simulink model "Hardware_With_Lead_Compensator"  (R2024b)
settings: Solver=FixedStepDiscrete  StartTime=0.0  StopTime=60  FixedStep=0.01  RelTol=1e-3  EnableMultiTasking=on
model workspace (MAT data in the model file):
  Kd = 0
  Ki = 0
  Kp = 0
libraries: arduinolib x3, cstblocks x1
settings Model: ExtModeTrigDuration=2  Creator=KSURCT General  LastModifiedBy=mafur
settings SolverCC: AlgebraicLoopSolver=TrustRegion  AutoInsertRateTranBlk=on
settings DataIOCC: ReturnWorkspaceOutputs=off
settings OptimizationCC: EnhancedBackFolding=on  PassReuseOutputArgsAs=Individual arguments  MaxStackSize=64  OptimizeBlockOrder=speed  DifferentSizesBufferReuse=on  EfficientTunableParamExpr=on
settings DebuggingCC: ParameterTunabilityLossMsg=error  UnconnectedInputMsg=warning  UnconnectedOutputMsg=warning  UnconnectedLineMsg=warning  ArithmeticOperatorsInVariantConditions=warning
settings HardwareCC: ProdBitPerPointer=32  ProdBitPerSizeT=32  ProdBitPerPtrDiffT=32  ProdLargestAtomicInteger=Long  ProdLargestAtomicFloat=Double  ProdWordSize=32  ProdHWDeviceType=ARM Compatible->ARM Cortex
settings ModelReferenceCC: EnableRefExpFcnMdlSchedulingChecks=on
settings SFSimCC: MATLABDynamicMemAlloc=off  CustomCodeUndefinedFunction=UseInterfaceOnly
settings RTWCC: Description=Embedded Coder  SystemTargetFile=ert.tlc  HardwareBoard=ESP32-WROOM(Arduino Compatible)  TLCOptions="-aInlineSetEventsForThisBaseRateFcn=TLC_FALSE -aSuppressMultiTaskScheduler=TLC_FALSE  -aRateBasedStepFcn=0"  TemplateMakefile=ert_default_tmf  GenerateReport=on  Toolchain=ESP32  BuildConfiguration=Faster Runs  IncludeHyperlinkInReport=on  LaunchReport=on  GenerateTraceInfo=on  GenerateTraceReport=on  GenerateTraceReportSl=on  GenerateTraceReportSf=on  GenerateTraceReportEml=on  GPUComputeCapability=3.5
settings CodeAppCC: ForceParamTrailComments=on  IgnoreCustomStorageClasses=off  OperatorAnnotations=on  SimulinkDataObjDesc=on  SFDataObjDesc=on  InsertBlockDesc=on
settings ERTTargetCC: SupportContinuousTime=on  SupportVariableSizeSignals=on  ExtModeTransport=3  ExtModeStaticAlloc=on  ExtModeAutomaticAllocSize=off  ExtModeStaticAllocSize=65536  ExtModeMexFile=ext_xcp  ExtModeIntrfLevel=Level2 - Open  InlinedParameterPlacement=Hierarchical  DynamicArrayContainerType=coder::array

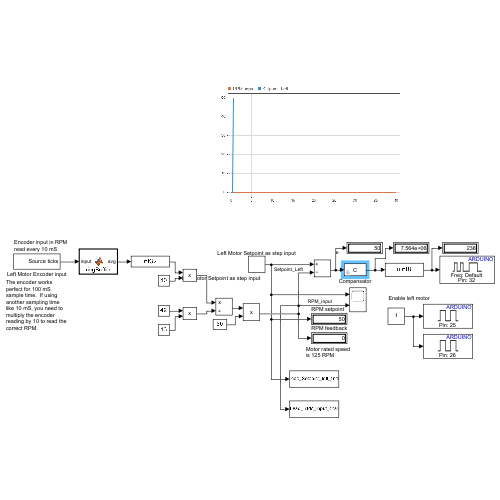
[thumbnail: Simulink's stored preview of the top-level diagram]
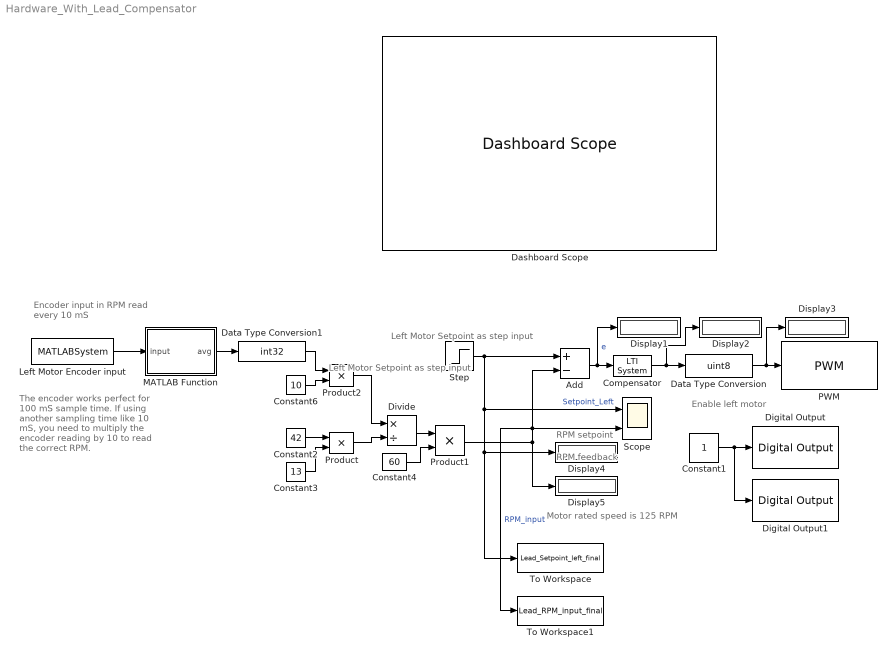
== system Hardware_With_Lead_Compensator ==
  note: RPM setpoint
  note: Left Motor Setpoint as step input
  note: Enable left motor
  note: RPM feedback
  note: Motor rated speed is 125 RPM
  note: Encoder input in RPM read every 10 mS
  note: The encoder works perfect for 100 mS sample time. If using another sampling time like 10 mS, you need to multiply the encoder reading by 10 to read the correct RPM.
  note: Left Motor Setpoint as step input
  Add : Sum  Inputs=+-
  Compensator : cstblocks/LTI System  sys=C  IC=[]  PadeOrder=0
  Constant1 : Constant
  Constant2 : Constant  Value=42
  Constant3 : Constant  Value=13
  Constant4 : Constant  Value=60
  Constant6 : Constant  Value=10
  Dashboard Scope : DashboardScope
  Data Type Conversion : DataTypeConversion  OutDataTypeStr=uint8  SaturateOnIntegerOverflow=off  RndMeth=Floor
  Data Type Conversion1 : DataTypeConversion  OutDataTypeStr=int32  SaturateOnIntegerOverflow=off  RndMeth=Floor
  Digital Output : arduinolib/Digital Output  pinNumber=25  Direction=output  blockPlatform=arduino
      settings: SourceProductName=Common
  Digital Output1 : arduinolib/Digital Output  pinNumber=26  Direction=output  blockPlatform=arduino
      settings: SourceProductName=Common
  Display{1..5} (5 alike) : Display
  Divide : Product  Inputs=*/
  Left Motor Encoder input : MATLABSystem  System=EncoderRead  pinA=int8(36)  pinB=int8(39)  id=int8(0)  SampleTime=0.01
      mask Type: EncoderRead
      mask Display:
      | disp('Source');
      | port_label('output',1,'ticks');
  MATLAB Function : MATLAB Function  TreatAsAtomicUnit=on
  PWM : arduinolib/PWM  pinNumber=32  frequencyType=Default  desiredFrequency=490.2  achievableFrequency=490.2
      settings: SourceProductName=Common
  Product : Product
  Product1 : Product
  Product2 : Product
  Scope : Scope  NumInputPorts=2
  Step : Step  Time=0.5  After=50  SampleTime=0
  To Workspace : ToWorkspace  VariableName=Lead_Setpoint_left_final  SaveFormat=Structure With Time  SampleTime=-1
  To Workspace1 : ToWorkspace  VariableName=Lead_RPM_input_final  SaveFormat=Structure With Time  SampleTime=-1
  wires:
  Left Motor Encoder input/1 -> MATLAB Function/1(input)
  Data Type Conversion/1 -> Display3/1, PWM/1
  Constant2/1 -> Product/1
  Constant3/1 -> Product/2
  Product/1 -> Divide/2
  Constant4/1 -> Product1/2
  Product1/1 -> Display5/1, Scope/2, To Workspace1/1, Add/2  "RPM_input"
  Step/1 -> Add/1, To Workspace/1, Display4/1, Scope/1  "Setpoint_Left"
  Add/1 -> Compensator/1, Display1/1  "e"
  Constant1/1 -> Digital Output1/1, Digital Output/1
  Divide/1 -> Product1/1
  Constant6/1 -> Product2/2
  Product2/1 -> Divide/1
  MATLAB Function/1(avg) -> Data Type Conversion1/1
  Data Type Conversion1/1 -> Product2/1
  Compensator/1 -> Display2/1, Data Type Conversion/1

== matlab function Hardware_With_Lead_Compensator/MATLAB Function ==
  data: input input; avg output
function avg = ringBuffer(input)
    % Define persistent variables
    persistent buffer index sum count;
    if isempty(buffer)
        buffer = zeros(1, 10); % Initialize buffer with 10 zeros
        index = 1; % Initialize index
        sum = 0; % Initialize sum
        count = 0; % Initialize count
    end
    
    % Update the buffer
    sum = sum - buffer(index); % Subtract the old value from sum
    new_input = double(input);
    buffer(index) = new_input; % Insert the new value
    sum = sum + new_input; % Add the new value to sum
    
    % Update the index
    index = index + 1;
    if index > 10
        index = 1; % Wrap around the index
    end
    
    % Update the count
    if  count < 10
        count = count + 1;
    end
    
    % Calculate the average
     avg = sum / count;
end
